simulink model "ex_blocchi_elementi_discreti"  (R2024b)
settings: Solver=VariableStepAuto  StartTime=0.0  StopTime=10.0  RelTol=1e-3
undefined symbols (not defined in the file): dspblkCoreblockFVToolHelper, gcbh

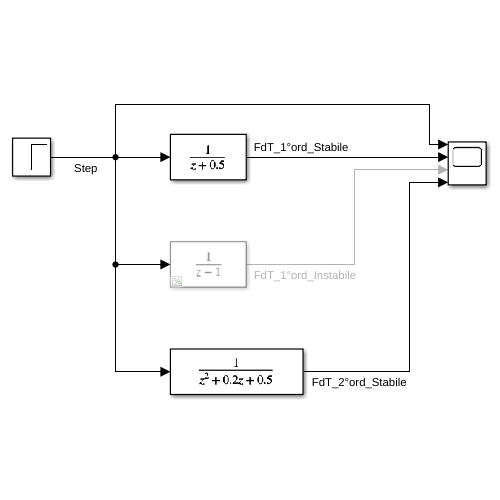
[thumbnail: Simulink's stored preview of the top-level diagram]
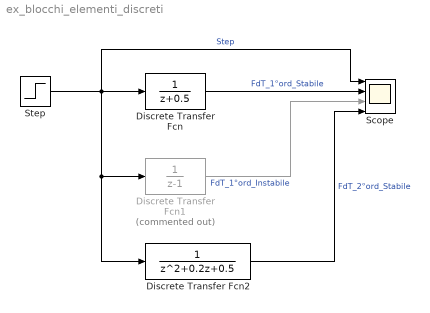
== system ex_blocchi_elementi_discreti ==
  Discrete Transfer Fcn : DiscreteTransferFcn
  Discrete Transfer Fcn1 : DiscreteTransferFcn  Commented=on  LoadFcn=dspblkCoreblockFVToolHelper(gcbh,'load');  Denominator=[1 -1]
      settings: CopyFcn=dspblkCoreblockFVToolHelper(gcbh,'copy');  DeleteFcn=dspblkCoreblockFVToolHelper(gcbh,'close');  ModelCloseFcn=dspblkCoreblockFVToolHelper(gcbh,'close');  PreSaveFcn=dspblkCoreblockFVToolHelper(gcbh,'presave');  PostSaveFcn=dspblkCoreblockFVToolHelper(gcbh,'postsave');  CloseFcn=dspblkCoreblockFVToolHelper(gcbh,'close');
  Discrete Transfer Fcn2 : DiscreteTransferFcn  LoadFcn=dspblkCoreblockFVToolHelper(gcbh,'load');  Denominator=[1 0.2 0.5]
      settings: CopyFcn=dspblkCoreblockFVToolHelper(gcbh,'copy');  DeleteFcn=dspblkCoreblockFVToolHelper(gcbh,'close');  ModelCloseFcn=dspblkCoreblockFVToolHelper(gcbh,'close');  PreSaveFcn=dspblkCoreblockFVToolHelper(gcbh,'presave');  PostSaveFcn=dspblkCoreblockFVToolHelper(gcbh,'postsave');  CloseFcn=dspblkCoreblockFVToolHelper(gcbh,'close');
  Scope : Scope  NumInputPorts=4
  Step : Step  SampleTime=0.01
  wires:
  Step/1 -> Discrete Transfer Fcn2/1, Discrete Transfer Fcn1/1, Scope/1, Discrete Transfer Fcn/1  "Step"
  Discrete Transfer Fcn/1 -> Scope/2  "FdT_1°ord_Stabile"
  Discrete Transfer Fcn1/1 -> Scope/3  "FdT_1°ord_Instabile"
  Discrete Transfer Fcn2/1 -> Scope/4  "FdT_2°ord_Stabile"
